simulink model "gm_UZ_EnDat"  (R2023b)
settings: Solver=FixedStepDiscrete  StartTime=0  StopTime=0.002  RelTol=1e-3
model workspace (MAT data in the model file):
  Select = 0
libraries: hdlsllib x314, hdlmdlgenlib x10, simulink x7, simulink_extras x3
(part 4 of 7)

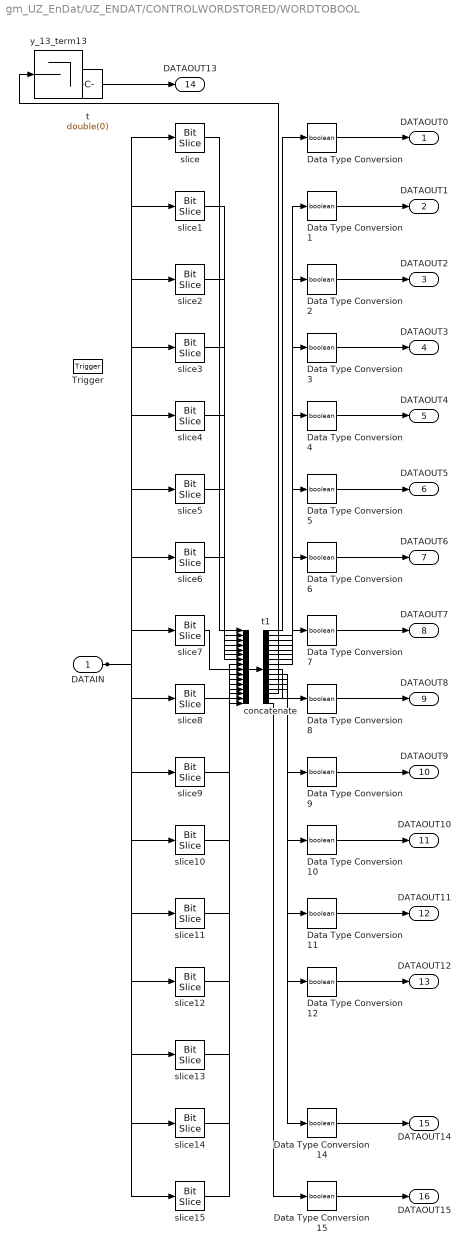
== system gm_UZ_EnDat/UZ_ENDAT/CONTROLWORDSTORED/WORDTOBOOL ==
  DATAIN : Inport  OutDataTypeStr=uint16  PortDimensions=1
  Trigger : TriggerPort  TriggerType=falling  VariantControl=(inherit)  OutputDataType=int8  InitialTriggerSignalState=positive  PortDimensions=1  OutDataTypeStr=boolean
  Data Type Conversion{,1..12,14..15} (15 alike) : DataTypeConversion  OutDataTypeStr=boolean  SaturateOnIntegerOverflow=off  RndMeth=Floor
  concatenate : Concatenate  NumInputs=16  Mode=Multidimensional array  ConcatenateDimension=2
  slice : hdlsllib/Logic and Bit Operations/Bit Slice  lidx=double(0)  ridx=double(0)
  slice1 : hdlsllib/Logic and Bit Operations/Bit Slice  lidx=double(1)  ridx=double(1)
  slice10 : hdlsllib/Logic and Bit Operations/Bit Slice  lidx=double(10)  ridx=double(10)
  slice11 : hdlsllib/Logic and Bit Operations/Bit Slice  lidx=double(11)  ridx=double(11)
  slice12 : hdlsllib/Logic and Bit Operations/Bit Slice  lidx=double(12)  ridx=double(12)
  slice13 : hdlsllib/Logic and Bit Operations/Bit Slice  lidx=double(13)  ridx=double(13)
  slice14 : hdlsllib/Logic and Bit Operations/Bit Slice  lidx=double(14)  ridx=double(14)
  slice15 : hdlsllib/Logic and Bit Operations/Bit Slice  lidx=double(15)  ridx=double(15)
  slice2 : hdlsllib/Logic and Bit Operations/Bit Slice  lidx=double(2)  ridx=double(2)
  slice3 : hdlsllib/Logic and Bit Operations/Bit Slice  lidx=double(3)  ridx=double(3)
  slice4 : hdlsllib/Logic and Bit Operations/Bit Slice  lidx=double(4)  ridx=double(4)
  slice5 : hdlsllib/Logic and Bit Operations/Bit Slice  lidx=double(5)  ridx=double(5)
  slice6 : hdlsllib/Logic and Bit Operations/Bit Slice  lidx=double(6)  ridx=double(6)
  slice7 : hdlsllib/Logic and Bit Operations/Bit Slice  lidx=double(7)  ridx=double(7)
  slice8 : hdlsllib/Logic and Bit Operations/Bit Slice  lidx=double(8)  ridx=double(8)
  slice9 : hdlsllib/Logic and Bit Operations/Bit Slice  lidx=double(9)  ridx=double(9)
  t : Constant  Value=double(0)  OutDataTypeStr=boolean  SampleTime=-1
  t1 : Demux  Outputs=16
  y_13_term13 : Terminator
  DATAOUT0 : Outport  InitialOutput=0
  DATAOUT1 : Outport  Port=2  InitialOutput=0
  DATAOUT2 : Outport  Port=3  InitialOutput=0
  DATAOUT3 : Outport  Port=4  InitialOutput=0
  DATAOUT4 : Outport  Port=5  InitialOutput=0
  DATAOUT5 : Outport  Port=6  InitialOutput=0
  DATAOUT6 : Outport  Port=7  InitialOutput=0
  DATAOUT7 : Outport  Port=8  InitialOutput=0
  DATAOUT8 : Outport  Port=9  InitialOutput=0
  DATAOUT9 : Outport  Port=10  InitialOutput=0
  DATAOUT10 : Outport  Port=11  InitialOutput=0
  DATAOUT11 : Outport  Port=12  InitialOutput=0
  DATAOUT12 : Outport  Port=13  InitialOutput=0
  DATAOUT13 : Outport  Port=14  InitialOutput=0
  DATAOUT14 : Outport  Port=15  InitialOutput=0
  DATAOUT15 : Outport  Port=16  InitialOutput=0
  wires:
  DATAIN/1 -> slice15/1, slice14/1, slice13/1, slice12/1, slice11/1, slice10/1, slice9/1, slice8/1, slice7/1, slice6/1, slice5/1, slice4/1, slice3/1, slice2/1, slice1/1, slice/1
  Data Type Conversion/1 -> DATAOUT0/1
  Data Type Conversion1/1 -> DATAOUT1/1
  Data Type Conversion10/1 -> DATAOUT10/1
  Data Type Conversion11/1 -> DATAOUT11/1
  Data Type Conversion12/1 -> DATAOUT12/1
  t/1 -> DATAOUT13/1
  Data Type Conversion14/1 -> DATAOUT14/1
  Data Type Conversion15/1 -> DATAOUT15/1
  Data Type Conversion2/1 -> DATAOUT2/1
  Data Type Conversion3/1 -> DATAOUT3/1
  Data Type Conversion4/1 -> DATAOUT4/1
  Data Type Conversion5/1 -> DATAOUT5/1
  Data Type Conversion6/1 -> DATAOUT6/1
  Data Type Conversion7/1 -> DATAOUT7/1
  Data Type Conversion8/1 -> DATAOUT8/1
  Data Type Conversion9/1 -> DATAOUT9/1
  concatenate/1 -> t1/1
  t1/1 -> Data Type Conversion/1
  t1/2 -> Data Type Conversion1/1
  t1/3 -> Data Type Conversion2/1
  t1/4 -> Data Type Conversion3/1
  t1/5 -> Data Type Conversion4/1
  t1/6 -> Data Type Conversion5/1
  t1/7 -> Data Type Conversion6/1
  t1/8 -> Data Type Conversion7/1
  t1/9 -> Data Type Conversion8/1
  t1/10 -> Data Type Conversion9/1
  t1/11 -> Data Type Conversion10/1
  t1/12 -> Data Type Conversion11/1
  t1/13 -> Data Type Conversion12/1
  t1/14 -> y_13_term13/1
  t1/15 -> Data Type Conversion14/1
  t1/16 -> Data Type Conversion15/1
  slice/1 -> concatenate/1
  slice1/1 -> concatenate/2
  slice2/1 -> concatenate/3
  slice3/1 -> concatenate/4
  slice4/1 -> concatenate/5
  slice5/1 -> concatenate/6
  slice6/1 -> concatenate/7
  slice7/1 -> concatenate/8
  slice8/1 -> concatenate/9
  slice9/1 -> concatenate/10
  slice10/1 -> concatenate/11
  slice11/1 -> concatenate/12
  slice12/1 -> concatenate/13
  slice13/1 -> concatenate/14
  slice14/1 -> concatenate/15
  slice15/1 -> concatenate/16

== system gm_UZ_EnDat/UZ_ENDAT/CRC_Check/DFF1 ==
  SET : Inport  OutDataTypeStr=boolean  PortDimensions=1  SampleTime=1e-08
  CLK : Inport  Port=2  OutDataTypeStr=boolean  PortDimensions=1  SampleTime=1e-08
  D : Inport  Port=3  OutDataTypeStr=boolean  PortDimensions=1  SampleTime=1e-08
  RST : Inport  Port=4  OutDataTypeStr=boolean  PortDimensions=1  SampleTime=1e-08
  JKFF : Subsystem
  NOT : Logic  Operator=NOT  Inputs=1  AllPortsSameDT=off  OutDataTypeStr=boolean  SampleTime=1e-08
  OQ : Outport  SampleTime=1e-08
  NOQ : Outport  Port=2  SampleTime=1e-08
  wires:
  SET/1 -> JKFF/1(SET)
  CLK/1 -> JKFF/2(CLK)
  D/1 -> NOT/1, JKFF/3(J)
  RST/1 -> JKFF/4(RST)
  JKFF/1(OQ) -> OQ/1
  JKFF/2(NOQ) -> NOQ/1
  NOT/1 -> JKFF/5(K)

== system gm_UZ_EnDat/UZ_ENDAT/CRC_Check/DFF2 ==
  SET : Inport  OutDataTypeStr=boolean  PortDimensions=1  SampleTime=1e-08
  CLK : Inport  Port=2  OutDataTypeStr=boolean  PortDimensions=1  SampleTime=1e-08
  D : Inport  Port=3  OutDataTypeStr=boolean  PortDimensions=1  SampleTime=1e-08
  RST : Inport  Port=4  OutDataTypeStr=boolean  PortDimensions=1  SampleTime=1e-08
  JKFF : Subsystem
  NOT : Logic  Operator=NOT  Inputs=1  AllPortsSameDT=off  OutDataTypeStr=boolean  SampleTime=1e-08
  OQ : Outport  SampleTime=1e-08
  NOQ : Outport  Port=2  SampleTime=1e-08
  wires:
  NOT/1 -> JKFF/5(K)
  JKFF/2(NOQ) -> NOQ/1
  JKFF/1(OQ) -> OQ/1
  RST/1 -> JKFF/4(RST)
  D/1 -> JKFF/3(J), NOT/1
  CLK/1 -> JKFF/2(CLK)
  SET/1 -> JKFF/1(SET)

== system gm_UZ_EnDat/UZ_ENDAT/CRC_Check/DFF3 ==
  SET : Inport  OutDataTypeStr=boolean  PortDimensions=1  SampleTime=1e-08
  CLK : Inport  Port=2  OutDataTypeStr=boolean  PortDimensions=1  SampleTime=1e-08
  D : Inport  Port=3  OutDataTypeStr=boolean  PortDimensions=1  SampleTime=1e-08
  RST : Inport  Port=4  OutDataTypeStr=boolean  PortDimensions=1  SampleTime=1e-08
  JKFF : Subsystem
  NOT : Logic  Operator=NOT  Inputs=1  AllPortsSameDT=off  OutDataTypeStr=boolean  SampleTime=1e-08
  OQ : Outport  SampleTime=1e-08
  NOQ : Outport  Port=2  SampleTime=1e-08
  wires:
  NOT/1 -> JKFF/5(K)
  JKFF/2(NOQ) -> NOQ/1
  JKFF/1(OQ) -> OQ/1
  RST/1 -> JKFF/4(RST)
  D/1 -> JKFF/3(J), NOT/1
  CLK/1 -> JKFF/2(CLK)
  SET/1 -> JKFF/1(SET)

== system gm_UZ_EnDat/UZ_ENDAT/CRC_Check/DFF4 ==
  SET : Inport  OutDataTypeStr=boolean  PortDimensions=1  SampleTime=1e-08
  CLK : Inport  Port=2  OutDataTypeStr=boolean  PortDimensions=1  SampleTime=1e-08
  D : Inport  Port=3  OutDataTypeStr=boolean  PortDimensions=1  SampleTime=1e-08
  RST : Inport  Port=4  OutDataTypeStr=boolean  PortDimensions=1  SampleTime=1e-08
  JKFF : Subsystem
  NOT : Logic  Operator=NOT  Inputs=1  AllPortsSameDT=off  OutDataTypeStr=boolean  SampleTime=1e-08
  OQ : Outport  SampleTime=1e-08
  NOQ : Outport  Port=2  SampleTime=1e-08
  wires:
  NOT/1 -> JKFF/5(K)
  JKFF/2(NOQ) -> NOQ/1
  JKFF/1(OQ) -> OQ/1
  RST/1 -> JKFF/4(RST)
  D/1 -> JKFF/3(J), NOT/1
  CLK/1 -> JKFF/2(CLK)
  SET/1 -> JKFF/1(SET)

== system gm_UZ_EnDat/UZ_ENDAT/CRC_Check/DFF5 ==
  SET : Inport  OutDataTypeStr=boolean  PortDimensions=1  SampleTime=1e-08
  CLK : Inport  Port=2  OutDataTypeStr=boolean  PortDimensions=1  SampleTime=1e-08
  D : Inport  Port=3  OutDataTypeStr=boolean  PortDimensions=1  SampleTime=1e-08
  RST : Inport  Port=4  OutDataTypeStr=boolean  PortDimensions=1  SampleTime=1e-08
  JKFF : Subsystem
  NOT : Logic  Operator=NOT  Inputs=1  AllPortsSameDT=off  OutDataTypeStr=boolean  SampleTime=1e-08
  OQ : Outport  SampleTime=1e-08
  NOQ : Outport  Port=2  SampleTime=1e-08
  wires:
  NOT/1 -> JKFF/5(K)
  JKFF/2(NOQ) -> NOQ/1
  JKFF/1(OQ) -> OQ/1
  RST/1 -> JKFF/4(RST)
  D/1 -> JKFF/3(J), NOT/1
  CLK/1 -> JKFF/2(CLK)
  SET/1 -> JKFF/1(SET)

== system gm_UZ_EnDat/UZ_ENDAT/INITIALOFF/CLKCNTER_FAST ==
  CLK : Inport  OutDataTypeStr=boolean  PortDimensions=1  SampleTime=1e-08
  Positional_Counter : Subsystem
  rd_0 : Delay  DelayLength=double(1)  InitialCondition=0  SampleTime=1e-08
  CNT : Outport  SampleTime=1e-08
  wires:
  Positional_Counter/1(divider) -> rd_0/1, CNT/1
  CLK/1 -> Positional_Counter/Trigger
  rd_0/1 -> Positional_Counter/1(valueout)

== system gm_UZ_EnDat/UZ_ENDAT/INITIALOFF/Subsystem6 ==
  FACTOR : Inport  OutMin=0  OutMax=60000  OutDataTypeStr=uint16  PortDimensions=1  SampleTime=1e-08
  Add1 : Sum  Inputs=+-  OutDataTypeStr=uint16  AccumDataTypeStr=fixdt(1, 17, 0)  RndMeth=Simplest  SaturateOnIntegerOverflow=on  SampleTime=1e-08
  Add2 : Sum  OutDataTypeStr=uint16  AccumDataTypeStr=fixdt(1, 33, 0)  RndMeth=Simplest  SaturateOnIntegerOverflow=on  SampleTime=1e-08
  Add3 : Sum  Inputs=+-  OutDataTypeStr=uint16  AccumDataTypeStr=fixdt(1, 17, 0)  RndMeth=Simplest  SaturateOnIntegerOverflow=on  SampleTime=1e-08
  Compare To Constant : Subsystem  mask(Compare To Constant){relop=<, const=double(100), OutDataTypeStr=boolean, ZeroCross=on}
      mask prompts: relop "Simulink:masks:Operator_MP"; const "Simulink:masks:ConstantValue_MP"; OutDataTypeStr "Simulink:masks:OutputDataType_MP"; ZeroCross "Simulink:masks:EnableZerocrossingDetection_MP"
      mask help: Simulink:masks:CompareToConstant_MD
      mask TypeOptions relop: == | ~= | < | <= | >= | >
      mask TypeOptions OutDataTypeStr: Simulink:masks:uint8 | Simulink:masks:boolean
      mask Callback ZeroCross: sl('zeroCrossEnable', gcbh);
      mask Display: disp(str)
  Constant : Constant  Value=20  OutDataTypeStr=int16  SampleTime=1e-08
  Constant1 : Constant  Value=-20  OutDataTypeStr=int16  SampleTime=1e-08
  Constant2 : Constant  Value=100  OutDataTypeStr=uint16  SampleTime=1e-08
  Constant3 : Constant  Value=2000  OutDataTypeStr=uint16  SampleTime=1e-08
  HwModeRegister : Delay  DelayLength=double(1)  InitialCondition=0  SampleTime=1e-08
  HwModeRegister1 : Delay  DelayLength=double(1)  InitialCondition=0  SampleTime=1e-08
  PipelineRegister : Delay  DelayLength=double(1)  InitialCondition=0  SampleTime=1e-08
  Product : Product  Inputs=**  OutDataTypeStr=int32  SampleTime=1e-08
  Switch : Switch  Criteria=u2 > Threshold  Threshold=double(0)  OutDataTypeStr=uint16  SampleTime=1e-08  SaturateOnIntegerOverflow=off  InputSameDT=off
  Switch1 : Switch  Criteria=u2 > Threshold  Threshold=double(0)  OutDataTypeStr=int16  SampleTime=1e-08  SaturateOnIntegerOverflow=off  InputSameDT=off
  out : Outport  SampleTime=1e-08
  wires:
  FACTOR/1 -> Add3/1, Add1/2, Compare To Constant/1(u)
  Add1/1 -> Switch/1
  Add2/1 -> out/1
  Add3/1 -> Switch/3
  Compare To Constant/1(y) -> Switch1/2, Switch/2
  Constant/1 -> Switch1/3
  Constant1/1 -> Switch1/1
  Constant2/1 -> Add3/2, Add1/1
  Constant3/1 -> Add2/1
  PipelineRegister/1 -> Add2/2
  Switch/1 -> HwModeRegister/1
  Switch1/1 -> HwModeRegister1/1
  Product/1 -> PipelineRegister/1
  HwModeRegister/1 -> Product/1
  HwModeRegister1/1 -> Product/2

== system gm_UZ_EnDat/UZ_ENDAT/ManualSerialize/Compare To Constant ==
  u : Inport  OutDataTypeStr=uint8  SampleTime=1e-08
  Compare : RelationalOperator  Operator===  OutDataTypeStr=boolean
  Constant : Constant  DisableCoverage=on  Value=const  OutDataTypeStr=Inherit: Inherit via back propagation  SampleTime=-1
  y : Outport  SampleTime=1e-08
  wires:
  u/1 -> Compare/1
  Compare/1 -> y/1
  Constant/1 -> Compare/2

== system gm_UZ_EnDat/UZ_ENDAT/ManualSerialize/Detect Increase1 ==
  note: U(k)
  note: Edge
  U : Inport  OutDataTypeStr=boolean  SampleTime=1e-08
  FixPt Relational Operator : RelationalOperator  Operator=>  OutDataTypeStr=boolean  SampleTime=1e-08  InputSameDT=off
  rd_0 : Delay  DelayLength=double(1)  InitialCondition=0  SampleTime=1e-08
  t : hdlmdlgenlib/Buffer
  Y : Outport  SampleTime=1e-08
  wires:
  U/1 -> t/1, FixPt Relational Operator/1
  t/1 -> rd_0/1
  FixPt Relational Operator/1 -> Y/1
  rd_0/1 -> FixPt Relational Operator/2

== system gm_UZ_EnDat/UZ_ENDAT/ManualSerialize/FF1 ==
  SET : Inport  OutDataTypeStr=boolean  PortDimensions=1  SampleTime=1e-08
  RST : Inport  Port=2  OutDataTypeStr=boolean  PortDimensions=1  SampleTime=1e-08
  S-R Flip-Flop : simulink_extras/Flip Flops/S-R Flip-Flop  initial_condition=0
  OQ : Outport  SampleTime=1e-08
  NOQ : Outport  Port=2  SampleTime=1e-08
  wires:
  SET/1 -> S-R Flip-Flop/1
  RST/1 -> S-R Flip-Flop/2
  S-R Flip-Flop/1 -> OQ/1
  S-R Flip-Flop/2 -> NOQ/1

== system gm_UZ_EnDat/UZ_ENDAT/ManualSerialize/SetZero64modified ==
  valin : Inport  OutDataTypeStr=fixdt(0, 64, 0)  PortDimensions=1
  setzero : Inport  Port=2  OutDataTypeStr=boolean  PortDimensions=1
  Trigger : TriggerPort  TriggerType=either  VariantControl=(inherit)  PortDimensions=1  OutDataTypeStr=boolean
  Constant2 : Constant  Value="fi(0,0,64,0,\"hex\",\"0000000000000000\")"  OutDataTypeStr=fixdt(0, 64, 0)  SampleTime=-1
  Index Vector1 : MultiPortSwitch  DataPortOrder=Zero-based contiguous  Inputs=2  DiagnosticForDefault=None  zeroidx=on  OutDataTypeStr=fixdt(0, 64, 0)  SaturateOnIntegerOverflow=off  InputSameDT=off
  valueout : Outport  InitialOutput=0  VectorParamsAs1DForOutWhenUnconnected=off
  wires:
  valin/1 -> Index Vector1/2
  setzero/1 -> Index Vector1/1
  Constant2/1 -> Index Vector1/3
  Index Vector1/1 -> valueout/1

== system gm_UZ_EnDat/UZ_ENDAT/ManualSerialize/Storage1 ==
  Data : Inport  OutDataTypeStr=fixdt(0, 64, 0)  PortDimensions=1  SampleTime=1e-08
  Write : Inport  Port=2  OutDataTypeStr=boolean  PortDimensions=1  SampleTime=1e-08
  Compare To Zero : Subsystem  mask(Compare To Zero){relop=>, OutDataTypeStr=boolean, ZeroCross=on}
      mask prompts: relop "Simulink:masks:Operator_MP"; OutDataTypeStr "Simulink:masks:OutputDataType_MP"; ZeroCross "Simulink:masks:EnableZerocrossingDetection_MP"
      mask help: Simulink:masks:CompareToZero_MD
      mask TypeOptions relop: == | ~= | < | <= | >= | >
      mask TypeOptions OutDataTypeStr: Simulink:masks:uint8 | Simulink:masks:boolean
      mask Callback ZeroCross: sl('zeroCrossEnable', gcbh);
      mask Display: disp([relop,' 0'])
  Logical Operator1 : Logic  AllPortsSameDT=off  OutDataTypeStr=boolean  SampleTime=1e-08
  out : Outport  SampleTime=1e-08
  wrok : Outport  Port=2  OutDataTypeStr=boolean  SampleTime=1e-08
  wires:
  Data/1 -> out/1, Compare To Zero/1(u)
  Write/1 -> Logical Operator1/1
  Compare To Zero/1(y) -> Logical Operator1/2
  Logical Operator1/1 -> wrok/1

== system gm_UZ_EnDat/UZ_ENDAT/ManualSerialize/Subsystem ==
  countclk : Inport  OutDataTypeStr=boolean  PortDimensions=1  SampleTime=1e-08
  reset : Inport  Port=2  OutDataTypeStr=boolean  PortDimensions=1  SampleTime=1e-08
  Detect Increase : Subsystem  mask(Detect Increase){vinit=double(0), InputProcessing=Elements as channels (sample based), OutDataTypeStr=boolean}
      mask prompts: vinit "Simulink:masks:InitialCondition_MP"; InputProcessing "Simulink:masks:InputProcessing_MP"; OutDataTypeStr "Simulink:masks:OutputDataType_MP"
      mask help: Simulink:masks:DetectIncrease_MD
      mask TypeOptions InputProcessing: Simulink:masks:ColumnsAsChannelsFrameBased | Simulink:masks:ElementsAsChannelsSampleBased
      mask TypeOptions OutDataTypeStr: Simulink:masks:uint8 | Simulink:masks:boolean
      mask Display: fprintf('U > U/z')
  HDL Counter_enbsw : Switch  Criteria=u2 ~= 0  Threshold=double(0)  OutDataTypeStr=uint8  SampleTime=1e-08  SaturateOnIntegerOverflow=off  InputSameDT=off
  adder : Sum  OutDataTypeStr=uint8  AccumDataTypeStr=uint8  SampleTime=1e-08
  compare : simulink/Logic and Bit Operations/Compare To Constant  relop===  const="fi(0,0,8,0,\"hex\",\"33\")"  OutDataTypeStr=boolean
  const : Constant  Value=0  VectorParams1D=off  OutDataTypeStr=uint8  SampleTime=1e-08
  countFrom : Constant  Value=0  VectorParams1D=off  OutDataTypeStr=uint8  SampleTime=1e-08
  rd_0 : Delay  DelayLength=double(1)  InitialCondition=0  SampleTime=1e-08
  rd_1 : Delay  DelayLength=double(2)  InitialCondition=0  SampleTime=1e-08
  rd_2 : Delay  DelayLength=double(1)  InitialCondition=0  SampleTime=1e-08
  stateControl : Constant  OutDataTypeStr=boolean  SampleTime=1e-08
  step_value : Constant  VectorParams1D=off  OutDataTypeStr=uint8  SampleTime=1e-08
  switch : Switch  Criteria=u2 ~= 0  Threshold=double(0)  OutDataTypeStr=uint8  SampleTime=1e-08  SaturateOnIntegerOverflow=off  InputSameDT=off
  switchEnable : MultiPortSwitch  DataPortOrder=Zero-based contiguous  Inputs=2  DiagnosticForDefault=None  zeroidx=on  OutDataTypeStr=uint8  SampleTime=1e-08  SaturateOnIntegerOverflow=off  InputSameDT=off
  switchReset : Switch  Criteria=u2 ~= 0  Threshold=double(0)  OutDataTypeStr=uint8  SampleTime=1e-08  SaturateOnIntegerOverflow=off  InputSameDT=off
  valin1 : Outport  SampleTime=1e-08  InitialOutput=0
  wires:
  countclk/1 -> Detect Increase/1(U)
  reset/1 -> rd_0/1
  stateControl/1 -> rd_1/1
  step_value/1 -> adder/2
  countFrom/1 -> switch/1
  Detect Increase/1(Y) -> switchEnable/1
  const/1 -> switchReset/1
  adder/1 -> switch/3
  compare/1 -> switch/2
  switch/1 -> switchEnable/3
  switchEnable/1 -> switchReset/3
  switchReset/1 -> HDL Counter_enbsw/1
  rd_0/1 -> switchReset/2
  rd_1/1 -> HDL Counter_enbsw/2
  HDL Counter_enbsw/1 -> rd_2/1
  rd_2/1 -> HDL Counter_enbsw/3, adder/1, compare/1, switchEnable/2, valin1/1

== system gm_UZ_EnDat/UZ_ENDAT/ManualSerialize/Triggered Subsystem ==
  DATA : Inport  OutDataTypeStr=boolean  PortDimensions=1
  valueout : Inport  Port=2  OutDataTypeStr=fixdt(0, 64, 0)  PortDimensions=1
  Trigger : TriggerPort  VariantControl=(inherit)  PortDimensions=1  OutDataTypeStr=boolean
  Bit Clear : simulink/Logic and Bit Operations/Bit Clear  iBit=double(50)
  Bit Set : simulink/Logic and Bit Operations/Bit Set  iBit=double(50)
  Bit Shift : hdlsllib/Logic and Bit Operations/Bit Shift  mode=Shift Right Logical  N=double(1)
  Switch : Switch  Criteria=u2 ~= 0  Threshold=double(0)  OutDataTypeStr=fixdt(0, 64, 0)  SaturateOnIntegerOverflow=off  InputSameDT=off
  valin : Outport  InitialOutput=0
  wires:
  DATA/1 -> Switch/2
  valueout/1 -> Bit Set/1, Bit Clear/1
  Bit Clear/1 -> Switch/3
  Bit Set/1 -> Switch/1
  Bit Shift/1 -> valin/1
  Switch/1 -> Bit Shift/1

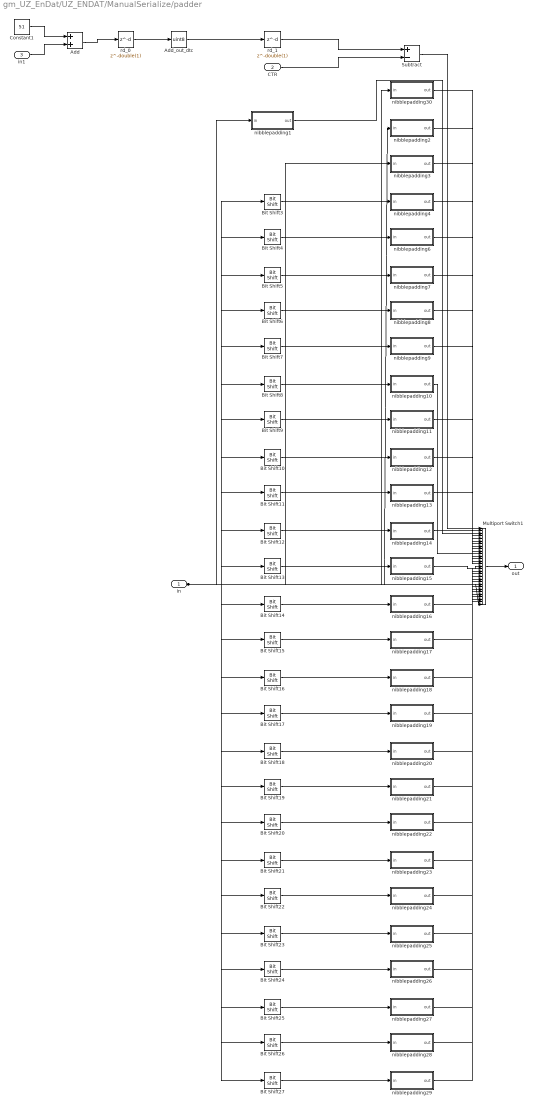
== system gm_UZ_EnDat/UZ_ENDAT/ManualSerialize/padder ==
  in : Inport  OutDataTypeStr=fixdt(0, 64, 0)  PortDimensions=1  SampleTime=1e-08
  CTR : Inport  Port=2  OutDataTypeStr=uint8  PortDimensions=1  SampleTime=1e-08
  in1 : Inport  Port=3  OutDataTypeStr=int8  PortDimensions=1  SampleTime=1e-08
  Add : Sum  OutDataTypeStr=fixdt(1, 10, 0)  AccumDataTypeStr=fixdt(1, 10, 0)  SampleTime=1e-08
  Add_out_dtc : DataTypeConversion  OutDataTypeStr=uint8  RndMeth=Simplest  SampleTime=1e-08  SaturateOnIntegerOverflow=off
  Bit Shift10 : hdlsllib/Logic and Bit Operations/Bit Shift  mode=Shift Right Logical  N=double(8)
  Bit Shift11 : hdlsllib/Logic and Bit Operations/Bit Shift  mode=Shift Right Logical  N=double(9)
  Bit Shift12 : hdlsllib/Logic and Bit Operations/Bit Shift  mode=Shift Right Logical  N=double(10)
  Bit Shift13 : hdlsllib/Logic and Bit Operations/Bit Shift  mode=Shift Right Logical  N=double(11)
  Bit Shift14 : hdlsllib/Logic and Bit Operations/Bit Shift  mode=Shift Right Logical  N=double(12)
  Bit Shift15 : hdlsllib/Logic and Bit Operations/Bit Shift  mode=Shift Right Logical  N=double(13)
  Bit Shift16 : hdlsllib/Logic and Bit Operations/Bit Shift  mode=Shift Right Logical  N=double(14)
  Bit Shift17 : hdlsllib/Logic and Bit Operations/Bit Shift  mode=Shift Right Logical  N=double(15)
  Bit Shift18 : hdlsllib/Logic and Bit Operations/Bit Shift  mode=Shift Right Logical  N=double(16)
  Bit Shift19 : hdlsllib/Logic and Bit Operations/Bit Shift  mode=Shift Right Logical  N=double(17)
  Bit Shift20 : hdlsllib/Logic and Bit Operations/Bit Shift  mode=Shift Right Logical  N=double(18)
  Bit Shift21 : hdlsllib/Logic and Bit Operations/Bit Shift  mode=Shift Right Logical  N=double(19)
  Bit Shift22 : hdlsllib/Logic and Bit Operations/Bit Shift  mode=Shift Right Logical  N=double(20)
  Bit Shift23 : hdlsllib/Logic and Bit Operations/Bit Shift  mode=Shift Right Logical  N=double(21)
  Bit Shift24 : hdlsllib/Logic and Bit Operations/Bit Shift  mode=Shift Right Logical  N=double(22)
  Bit Shift25 : hdlsllib/Logic and Bit Operations/Bit Shift  mode=Shift Right Logical  N=double(23)
  Bit Shift26 : hdlsllib/Logic and Bit Operations/Bit Shift  mode=Shift Right Logical  N=double(24)
  Bit Shift27 : hdlsllib/Logic and Bit Operations/Bit Shift  mode=Shift Right Logical  N=double(25)
  Bit Shift3 : hdlsllib/Logic and Bit Operations/Bit Shift  mode=Shift Right Logical  N=double(1)
  Bit Shift4 : hdlsllib/Logic and Bit Operations/Bit Shift  mode=Shift Right Logical  N=double(2)
  Bit Shift5 : hdlsllib/Logic and Bit Operations/Bit Shift  mode=Shift Right Logical  N=double(3)
  Bit Shift6 : hdlsllib/Logic and Bit Operations/Bit Shift  mode=Shift Right Logical  N=double(4)
  Bit Shift7 : hdlsllib/Logic and Bit Operations/Bit Shift  mode=Shift Right Logical  N=double(5)
  Bit Shift8 : hdlsllib/Logic and Bit Operations/Bit Shift  mode=Shift Right Logical  N=double(6)
  Bit Shift9 : hdlsllib/Logic and Bit Operations/Bit Shift  mode=Shift Right Logical  N=double(7)
  Constant1 : Constant  Value=51  OutDataTypeStr=uint8  SampleTime=1e-08
  Multiport Switch1 : MultiPortSwitch  DataPortOrder=Zero-based contiguous  Inputs=29  DataPortForDefault=Additional data port  DiagnosticForDefault=None  zeroidx=on  OutDataTypeStr=fixdt(0, 64, 0)  RndMeth=Simplest  SampleTime=1e-08  SaturateOnIntegerOverflow=off  InputSameDT=off
  Subtract : Sum  Inputs=+-  OutDataTypeStr=uint8  AccumDataTypeStr=fixdt(1, 9, 0)  RndMeth=Simplest  SaturateOnIntegerOverflow=on  SampleTime=1e-08
  nibblepadding1 : Subsystem
  nibblepadding10 : Subsystem
  nibblepadding11 : Subsystem
  nibblepadding12 : Subsystem
  nibblepadding13 : Subsystem
  nibblepadding14 : Subsystem
  nibblepadding15 : Subsystem
  nibblepadding16 : Subsystem
  nibblepadding17 : Subsystem
  nibblepadding18 : Subsystem
  nibblepadding19 : Subsystem
  nibblepadding2 : Subsystem
  nibblepadding20 : Subsystem
  nibblepadding21 : Subsystem
  nibblepadding22 : Subsystem
  nibblepadding23 : Subsystem
  nibblepadding24 : Subsystem
  nibblepadding25 : Subsystem
  nibblepadding26 : Subsystem
  nibblepadding27 : Subsystem
  nibblepadding28 : Subsystem
  nibblepadding29 : Subsystem
  nibblepadding3 : Subsystem
  nibblepadding30 : Subsystem
  nibblepadding4 : Subsystem
  nibblepadding6 : Subsystem
  nibblepadding7 : Subsystem
  nibblepadding8 : Subsystem
  nibblepadding9 : Subsystem
  rd_0 : Delay  DelayLength=double(1)  InitialCondition=0  SampleTime=1e-08
  rd_1 : Delay  DelayLength=double(1)  InitialCondition=0  SampleTime=1e-08
  out : Outport  SampleTime=1e-08
  wires:
  in/1 -> Multiport Switch1/31, Bit Shift9/1, Bit Shift8/1, Bit Shift7/1, Bit Shift6/1, Bit Shift5/1, Bit Shift4/1, Bit Shift3/1, Bit Shift27/1, Bit Shift26/1, Bit Shift25/1, Bit Shift24/1, Bit Shift23/1, Bit Shift22/1, Bit Shift21/1, Bit Shift20/1, Bit Shift19/1, Bit Shift18/1, Bit Shift17/1, Bit Shift16/1, Bit Shift15/1, Bit Shift14/1, Bit Shift13/1, Bit Shift12/1, Bit Shift11/1, Bit Shift10/1, nibblepadding1/1(in), nibblepadding2/1(in), nibblepadding3/1(in), nibblepadding30/1(in)
  CTR/1 -> Subtract/2
  in1/1 -> Add/2
  Bit Shift10/1 -> nibblepadding12/1(in)
  Bit Shift11/1 -> nibblepadding13/1(in)
  Bit Shift12/1 -> nibblepadding14/1(in)
  Bit Shift13/1 -> nibblepadding15/1(in)
  Bit Shift14/1 -> nibblepadding16/1(in)
  Bit Shift15/1 -> nibblepadding17/1(in)
  Bit Shift16/1 -> nibblepadding18/1(in)
  Bit Shift17/1 -> nibblepadding19/1(in)
  Bit Shift18/1 -> nibblepadding20/1(in)
  Bit Shift19/1 -> nibblepadding21/1(in)
  Bit Shift20/1 -> nibblepadding22/1(in)
  Bit Shift21/1 -> nibblepadding23/1(in)
  Bit Shift22/1 -> nibblepadding24/1(in)
  Bit Shift23/1 -> nibblepadding25/1(in)
  Bit Shift24/1 -> nibblepadding26/1(in)
  Bit Shift25/1 -> nibblepadding27/1(in)
  Bit Shift26/1 -> nibblepadding28/1(in)
  Bit Shift27/1 -> nibblepadding29/1(in)
  Bit Shift3/1 -> nibblepadding4/1(in)
  Bit Shift4/1 -> nibblepadding6/1(in)
  Bit Shift5/1 -> nibblepadding7/1(in)
  Bit Shift6/1 -> nibblepadding8/1(in)
  Bit Shift7/1 -> nibblepadding9/1(in)
  Bit Shift8/1 -> nibblepadding10/1(in)
  Bit Shift9/1 -> nibblepadding11/1(in)
  Constant1/1 -> Add/1
  Multiport Switch1/1 -> out/1
  Subtract/1 -> Multiport Switch1/1
  nibblepadding1/1(out) -> Multiport Switch1/3
  nibblepadding10/1(out) -> Multiport Switch1/11
  nibblepadding11/1(out) -> Multiport Switch1/12
  nibblepadding12/1(out) -> Multiport Switch1/13
  nibblepadding13/1(out) -> Multiport Switch1/14
  nibblepadding14/1(out) -> Multiport Switch1/15
  nibblepadding15/1(out) -> Multiport Switch1/16
  nibblepadding16/1(out) -> Multiport Switch1/17
  nibblepadding17/1(out) -> Multiport Switch1/18
  nibblepadding18/1(out) -> Multiport Switch1/19
  nibblepadding19/1(out) -> Multiport Switch1/20
  nibblepadding2/1(out) -> Multiport Switch1/4
  nibblepadding20/1(out) -> Multiport Switch1/21
  nibblepadding21/1(out) -> Multiport Switch1/22
  nibblepadding22/1(out) -> Multiport Switch1/23
  nibblepadding23/1(out) -> Multiport Switch1/24
  nibblepadding24/1(out) -> Multiport Switch1/25
  nibblepadding25/1(out) -> Multiport Switch1/26
  nibblepadding26/1(out) -> Multiport Switch1/27
  nibblepadding27/1(out) -> Multiport Switch1/28
  nibblepadding28/1(out) -> Multiport Switch1/29
  nibblepadding29/1(out) -> Multiport Switch1/30
  nibblepadding3/1(out) -> Multiport Switch1/5
  nibblepadding30/1(out) -> Multiport Switch1/2
  nibblepadding4/1(out) -> Multiport Switch1/6
  nibblepadding6/1(out) -> Multiport Switch1/7
  nibblepadding7/1(out) -> Multiport Switch1/8
  nibblepadding8/1(out) -> Multiport Switch1/9
  nibblepadding9/1(out) -> Multiport Switch1/10
  Add/1 -> rd_0/1
  Add_out_dtc/1 -> rd_1/1
  rd_1/1 -> Subtract/1
  rd_0/1 -> Add_out_dtc/1

== system gm_UZ_EnDat/UZ_ENDAT/RESPONSESLICER3X/19BITSLICER ==
  DATA : Inport  OutDataTypeStr=fixdt(0, 64, 0)  PortDimensions=1  SampleTime=1e-08
  DATA1 : Inport  Port=2  OutDataTypeStr=fixdt(0, 64, 0)  PortDimensions=1  SampleTime=1e-08
  DATA2 : Inport  Port=3  OutDataTypeStr=fixdt(0, 64, 0)  PortDimensions=1  SampleTime=1e-08
  Enable : EnablePort  OutDataTypeStr=boolean
  responseslicer : Subsystem
  responseslicer1 : Subsystem
  responseslicer1_term2 : Terminator
  responseslicer2 : Subsystem
  responseslicer2_term2 : Terminator
  CRC : Outport  SampleTime=1e-08  InitialOutput=0
  payload : Outport  Port=2  SampleTime=1e-08  InitialOutput=0
  CRC1 : Outport  Port=3  SampleTime=1e-08  InitialOutput=0
  payload1 : Outport  Port=4  SampleTime=1e-08  InitialOutput=0
  CRC2 : Outport  Port=5  SampleTime=1e-08  InitialOutput=0
  payload2 : Outport  Port=6  SampleTime=1e-08  InitialOutput=0
  sensorerror : Outport  Port=7  SampleTime=1e-08  InitialOutput=0
  wires:
  DATA/1 -> responseslicer/1(DATA)
  DATA1/1 -> responseslicer1/1(DATA)
  DATA2/1 -> responseslicer2/1(DATA)
  responseslicer/1(CRC) -> CRC/1
  responseslicer/2(payload) -> payload/1
  responseslicer/3(error) -> sensorerror/1
  responseslicer1/1(CRC) -> CRC1/1
  responseslicer1/2(payload) -> payload1/1
  responseslicer1/3(error) -> responseslicer1_term2/1
  responseslicer2/1(CRC) -> CRC2/1
  responseslicer2/2(payload) -> payload2/1
  responseslicer2/3(error) -> responseslicer2_term2/1

== system gm_UZ_EnDat/UZ_ENDAT/RESPONSESLICER3X/21BITSLICER ==
  DATA : Inport  OutDataTypeStr=fixdt(0, 64, 0)  PortDimensions=1  SampleTime=1e-08
  DATA1 : Inport  Port=2  OutDataTypeStr=fixdt(0, 64, 0)  PortDimensions=1  SampleTime=1e-08
  DATA2 : Inport  Port=3  OutDataTypeStr=fixdt(0, 64, 0)  PortDimensions=1  SampleTime=1e-08
  Enable : EnablePort  OutDataTypeStr=boolean
  responseslicer : Subsystem
  responseslicer3 : Subsystem
  responseslicer3_term2 : Terminator
  responseslicer4 : Subsystem
  responseslicer4_term2 : Terminator
  CRC : Outport  SampleTime=1e-08  InitialOutput=0
  payload : Outport  Port=2  SampleTime=1e-08  InitialOutput=0
  CRC1 : Outport  Port=3  SampleTime=1e-08  InitialOutput=0
  payload1 : Outport  Port=4  SampleTime=1e-08  InitialOutput=0
  CRC2 : Outport  Port=5  SampleTime=1e-08  InitialOutput=0
  payload2 : Outport  Port=6  SampleTime=1e-08  InitialOutput=0
  sensorerror : Outport  Port=7  SampleTime=1e-08  InitialOutput=0
  wires:
  DATA/1 -> responseslicer/1(DATA)
  DATA1/1 -> responseslicer4/1(DATA)
  DATA2/1 -> responseslicer3/1(DATA)
  responseslicer/1(CRC) -> CRC/1
  responseslicer/2(payload) -> payload/1
  responseslicer/3(error) -> sensorerror/1
  responseslicer3/1(CRC) -> CRC2/1
  responseslicer3/2(payload) -> payload2/1
  responseslicer3/3(error) -> responseslicer3_term2/1
  responseslicer4/1(CRC) -> CRC1/1
  responseslicer4/2(payload) -> payload1/1
  responseslicer4/3(error) -> responseslicer4_term2/1

== system gm_UZ_EnDat/UZ_ENDAT/RESPONSESLICER3X/23BITSLICER ==
  DATA : Inport  OutDataTypeStr=fixdt(0, 64, 0)  PortDimensions=1  SampleTime=1e-08
  DATA1 : Inport  Port=2  OutDataTypeStr=fixdt(0, 64, 0)  PortDimensions=1  SampleTime=1e-08
  DATA2 : Inport  Port=3  OutDataTypeStr=fixdt(0, 64, 0)  PortDimensions=1  SampleTime=1e-08
  Enable : EnablePort  OutDataTypeStr=boolean
  responseslicer : Subsystem
  responseslicer1 : Subsystem
  responseslicer1_term2 : Terminator
  responseslicer2 : Subsystem
  responseslicer2_term2 : Terminator
  CRC : Outport  SampleTime=1e-08  InitialOutput=0
  payload : Outport  Port=2  SampleTime=1e-08  InitialOutput=0
  CRC1 : Outport  Port=3  SampleTime=1e-08  InitialOutput=0
  payload1 : Outport  Port=4  SampleTime=1e-08  InitialOutput=0
  CRC2 : Outport  Port=5  SampleTime=1e-08  InitialOutput=0
  payload2 : Outport  Port=6  SampleTime=1e-08  InitialOutput=0
  sensorerror : Outport  Port=7  SampleTime=1e-08  InitialOutput=0
  wires:
  DATA/1 -> responseslicer/1(DATA)
  DATA1/1 -> responseslicer1/1(DATA)
  DATA2/1 -> responseslicer2/1(DATA)
  responseslicer/1(CRC) -> CRC/1
  responseslicer/2(payload) -> payload/1
  responseslicer/3(error) -> sensorerror/1
  responseslicer1/1(CRC) -> CRC1/1
  responseslicer1/2(payload) -> payload1/1
  responseslicer1/3(error) -> responseslicer1_term2/1
  responseslicer2/1(CRC) -> CRC2/1
  responseslicer2/2(payload) -> payload2/1
  responseslicer2/3(error) -> responseslicer2_term2/1

== system gm_UZ_EnDat/UZ_ENDAT/RESPONSESLICER3X/25BITSLICER ==
  DATA : Inport  OutDataTypeStr=fixdt(0, 64, 0)  PortDimensions=1  SampleTime=1e-08
  DATA1 : Inport  Port=2  OutDataTypeStr=fixdt(0, 64, 0)  PortDimensions=1  SampleTime=1e-08
  DATA2 : Inport  Port=3  OutDataTypeStr=fixdt(0, 64, 0)  PortDimensions=1  SampleTime=1e-08
  Enable : EnablePort  OutDataTypeStr=boolean
  responseslicer : Subsystem
  responseslicer1 : Subsystem
  responseslicer1_term2 : Terminator
  responseslicer2 : Subsystem
  responseslicer2_term2 : Terminator
  CRC : Outport  SampleTime=1e-08  InitialOutput=0
  payload : Outport  Port=2  SampleTime=1e-08  InitialOutput=0
  CRC1 : Outport  Port=3  SampleTime=1e-08  InitialOutput=0
  payload1 : Outport  Port=4  SampleTime=1e-08  InitialOutput=0
  CRC2 : Outport  Port=5  SampleTime=1e-08  InitialOutput=0
  payload2 : Outport  Port=6  SampleTime=1e-08  InitialOutput=0
  sensorerror : Outport  Port=7  SampleTime=1e-08  InitialOutput=0
  wires:
  DATA/1 -> responseslicer/1(DATA)
  DATA1/1 -> responseslicer1/1(DATA)
  DATA2/1 -> responseslicer2/1(DATA)
  responseslicer/1(CRC) -> CRC/1
  responseslicer/2(payload) -> payload/1
  responseslicer/3(error) -> sensorerror/1
  responseslicer1/1(CRC) -> CRC1/1
  responseslicer1/2(payload) -> payload1/1
  responseslicer1/3(error) -> responseslicer1_term2/1
  responseslicer2/1(CRC) -> CRC2/1
  responseslicer2/2(payload) -> payload2/1
  responseslicer2/3(error) -> responseslicer2_term2/1

== system gm_UZ_EnDat/UZ_ENDAT/RESPONSESLICER3X/27BITSLICER ==
  DATA : Inport  OutDataTypeStr=fixdt(0, 64, 0)  PortDimensions=1  SampleTime=1e-08
  DATA1 : Inport  Port=2  OutDataTypeStr=fixdt(0, 64, 0)  PortDimensions=1  SampleTime=1e-08
  DATA2 : Inport  Port=3  OutDataTypeStr=fixdt(0, 64, 0)  PortDimensions=1  SampleTime=1e-08
  Enable : EnablePort  OutDataTypeStr=boolean
  responseslicer : Subsystem
  responseslicer1 : Subsystem
  responseslicer1_term2 : Terminator
  responseslicer2 : Subsystem
  responseslicer2_term2 : Terminator
  CRC : Outport  SampleTime=1e-08  InitialOutput=0
  payload : Outport  Port=2  SampleTime=1e-08  InitialOutput=0
  CRC1 : Outport  Port=3  SampleTime=1e-08  InitialOutput=0
  payload1 : Outport  Port=4  SampleTime=1e-08  InitialOutput=0
  CRC2 : Outport  Port=5  SampleTime=1e-08  InitialOutput=0
  payload2 : Outport  Port=6  SampleTime=1e-08  InitialOutput=0
  sensorerror : Outport  Port=7  SampleTime=1e-08  InitialOutput=0
  wires:
  DATA/1 -> responseslicer/1(DATA)
  DATA1/1 -> responseslicer1/1(DATA)
  DATA2/1 -> responseslicer2/1(DATA)
  responseslicer/1(CRC) -> CRC/1
  responseslicer/2(payload) -> payload/1
  responseslicer/3(error) -> sensorerror/1
  responseslicer1/1(CRC) -> CRC1/1
  responseslicer1/2(payload) -> payload1/1
  responseslicer1/3(error) -> responseslicer1_term2/1
  responseslicer2/1(CRC) -> CRC2/1
  responseslicer2/2(payload) -> payload2/1
  responseslicer2/3(error) -> responseslicer2_term2/1

== system gm_UZ_EnDat/UZ_ENDAT/Storage16/Compare To Zero ==
  u : Inport  OutDataTypeStr=uint16  SampleTime=1e-08
  Compare : RelationalOperator  Operator===  OutDataTypeStr=boolean  SampleTime=1e-08
  Constant : Constant  Value=0  OutDataTypeStr=uint16  SampleTime=1e-08
  y : Outport  SampleTime=1e-08
  wires:
  u/1 -> Compare/1
  Compare/1 -> y/1
  Constant/1 -> Compare/2

== system gm_UZ_EnDat/UZ_ENDAT/Subsystem2/ManualDeserializere ==
  CLK : Inport  OutDataTypeStr=boolean  PortDimensions=1  SampleTime=1e-08
  SLOWCLCK : Inport  Port=2  OutDataTypeStr=boolean  PortDimensions=1  SampleTime=1e-08
  DATA : Inport  Port=3  OutDataTypeStr=uint16  PortDimensions=1  SampleTime=1e-08
  reset : Inport  Port=4  OutDataTypeStr=boolean  PortDimensions=1  SampleTime=1e-08
  Constant3 : Constant  Value=0  OutDataTypeStr=boolean  SampleTime=1e-08
  Delay1 : Delay  DelayLength=double(1)  InitialCondition=0
  Multiport Switch : MultiPortSwitch  Inputs=6  DataPortForDefault=Additional data port  DiagnosticForDefault=None  SampleTime=1e-08  SaturateOnIntegerOverflow=off  InputSameDT=off
  WORDTOBOOL : Subsystem
  WORDTOBOOL_term{6..15} (10 alike) : Terminator
  ramwatcher : Subsystem
  valin : Outport  SampleTime=1e-08  InitialOutput=0
  wires:
  CLK/1 -> WORDTOBOOL/Trigger
  DATA/1 -> WORDTOBOOL/1(DATAIN)
  Constant3/1 -> Multiport Switch/8
  Multiport Switch/1 -> valin/1
  WORDTOBOOL/1(DATAOUT0) -> Multiport Switch/7
  WORDTOBOOL/2(DATAOUT1) -> Multiport Switch/6
  WORDTOBOOL/3(DATAOUT2) -> Multiport Switch/5
  WORDTOBOOL/4(DATAOUT3) -> Multiport Switch/4
  WORDTOBOOL/5(DATAOUT4) -> Multiport Switch/3
  WORDTOBOOL/6(DATAOUT5) -> Multiport Switch/2
  ramwatcher/1(SEL) -> Multiport Switch/1, Delay1/1
  WORDTOBOOL/7(DATAOUT6) -> WORDTOBOOL_term6/1
  WORDTOBOOL/8(DATAOUT7) -> WORDTOBOOL_term7/1
  WORDTOBOOL/9(DATAOUT8) -> WORDTOBOOL_term8/1
  WORDTOBOOL/10(DATAOUT9) -> WORDTOBOOL_term9/1
  WORDTOBOOL/11(DATAOUT10) -> WORDTOBOOL_term10/1
  WORDTOBOOL/12(DATAOUT11) -> WORDTOBOOL_term11/1
  WORDTOBOOL/13(DATAOUT12) -> WORDTOBOOL_term12/1
  WORDTOBOOL/14(DATAOUT13) -> WORDTOBOOL_term13/1
  WORDTOBOOL/15(DATAOUT14) -> WORDTOBOOL_term14/1
  WORDTOBOOL/16(DATAOUT15) -> WORDTOBOOL_term15/1
  Delay1/1 -> ramwatcher/1(In1)
  reset/1 -> ramwatcher/2(reset)
  SLOWCLCK/1 -> ramwatcher/Trigger

== system gm_UZ_EnDat/UZ_ENDAT/ageprovider/Detect Increase1 ==
  note: U(k)
  note: Edge
  U : Inport  OutDataTypeStr=boolean  SampleTime=1e-08
  FixPt Relational Operator : RelationalOperator  Operator=>  OutDataTypeStr=boolean  SampleTime=1e-08  InputSameDT=off
  rd_0 : Delay  DelayLength=double(1)  InitialCondition=0  SampleTime=1e-08
  t : hdlmdlgenlib/Buffer
  Y : Outport  SampleTime=1e-08
  wires:
  U/1 -> t/1, FixPt Relational Operator/1
  t/1 -> rd_0/1
  FixPt Relational Operator/1 -> Y/1
  rd_0/1 -> FixPt Relational Operator/2

== system gm_UZ_EnDat/UZ_ENDAT/ramselektor/Increment Stored Integer ==
  u : Inport  OutDataTypeStr=fixdt(0, 4, 0)
  FixPt Constant : Constant  OutDataTypeStr=fixdt(0, 4, 0)  SampleTime=-1
  FixPt Data Type Duplicate : DataTypeDuplicate  DisableCoverage=on  NumInputPorts=3
  FixPt Gateway In : DataTypeConversion  OutDataTypeStr=fixdt(0,4,0)
  FixPt Sum1 : Sum  OutDataTypeStr=fixdt(0, 4, 0)  AccumDataTypeStr=fixdt(0, 5, 0)
  sigspec : SignalSpecification  OutDataTypeStr=fixdt(0, 4, 0)  Dimensions=1
  y : Outport  InitialOutput=0
  wires:
  u/1 -> FixPt Sum1/1, FixPt Data Type Duplicate/2
  FixPt Constant/1 -> sigspec/1
  FixPt Gateway In/1 -> FixPt Sum1/2, FixPt Data Type Duplicate/3
  FixPt Sum1/1 -> FixPt Data Type Duplicate/1, y/1
  sigspec/1 -> FixPt Gateway In/1

== system gm_UZ_EnDat/UZ_ENDAT/signalquality/Detect Increase1 ==
  note: U(k)
  note: Edge
  U : Inport  OutDataTypeStr=boolean  SampleTime=1e-08
  FixPt Relational Operator : RelationalOperator  Operator=>  OutDataTypeStr=boolean  SampleTime=1e-08  InputSameDT=off
  rd_0 : Delay  DelayLength=double(1)  InitialCondition=0  SampleTime=1e-08
  t : hdlmdlgenlib/Buffer
  Y : Outport  SampleTime=1e-08
  wires:
  U/1 -> t/1, FixPt Relational Operator/1
  t/1 -> rd_0/1
  FixPt Relational Operator/1 -> Y/1
  rd_0/1 -> FixPt Relational Operator/2

== system gm_UZ_EnDat/UZ_ENDAT/timingprovider/CLKCNTER_POSCNTR ==
  CLK : Inport  OutDataTypeStr=boolean  PortDimensions=1  SampleTime=1e-08
  CLK2CNT : Inport  Port=2  OutDataTypeStr=boolean  PortDimensions=1  SampleTime=1e-08
  ResetCNT : Inport  Port=3  OutDataTypeStr=boolean  PortDimensions=1  SampleTime=1e-08
  Delay1 : Delay  DelayLength=double(1)  InitialCondition=0  SampleTime=1e-08
  Delay1_enbsw : Switch  Criteria=u2 ~= 0  Threshold=double(0)  OutDataTypeStr=uint32  SampleTime=1e-08  SaturateOnIntegerOverflow=off  InputSameDT=off
  Positional_Counter : Subsystem
  SetZero32modified : Subsystem
  SetZero32modified1 : Subsystem
  delayMatch : Delay  DelayLength=double(2)  InitialCondition=0  SampleTime=1e-08
  delayMatch1 : Delay  DelayLength=double(2)  InitialCondition=0  SampleTime=1e-08
  delayMatch2 : Delay  DelayLength=double(2)  InitialCondition=0  SampleTime=1e-08
  stateControl : Constant  OutDataTypeStr=boolean  SampleTime=1e-08
  CNT : Outport  SampleTime=1e-08
  wires:
  CLK/1 -> delayMatch/1
  CLK2CNT/1 -> delayMatch1/1
  stateControl/1 -> delayMatch2/1
  delayMatch2/1 -> Delay1_enbsw/2
  ResetCNT/1 -> SetZero32modified/2(setzero), SetZero32modified1/2(setzero)
  delayMatch/1 -> SetZero32modified/Trigger, SetZero32modified1/Trigger
  delayMatch1/1 -> Positional_Counter/Trigger
  SetZero32modified1/1(valueout) -> Positional_Counter/1(valueout)
  Positional_Counter/1(divider) -> SetZero32modified/1(valin)
  Delay1/1 -> Delay1_enbsw/3, SetZero32modified1/1(valin), CNT/1
  SetZero32modified/1(valueout) -> Delay1_enbsw/1
  Delay1_enbsw/1 -> Delay1/1

== system gm_UZ_EnDat/UZ_ENDAT/timingprovider/CLKCNTER_POSCNTR1 ==
  CLK : Inport  OutDataTypeStr=boolean  PortDimensions=1  SampleTime=1e-08
  CLK2CNT : Inport  Port=2  OutDataTypeStr=boolean  PortDimensions=1  SampleTime=1e-08
  ResetCNT : Inport  Port=3  OutDataTypeStr=boolean  PortDimensions=1  SampleTime=1e-08
  Delay1_enbsw : Switch  Criteria=u2 ~= 0  Threshold=double(0)  OutDataTypeStr=uint32  SampleTime=1e-08  SaturateOnIntegerOverflow=off  InputSameDT=off
  Positional_Counter : Subsystem
  SetZero32modified : Subsystem
  rd_0 : Delay  DelayLength=double(2)  InitialCondition=0  SampleTime=1e-08
  rd_1 : Delay  DelayLength=double(1)  InitialCondition=0  SampleTime=1e-08
  stateControl : Constant  OutDataTypeStr=boolean  SampleTime=1e-08
  CNT : Outport  SampleTime=1e-08
  wires:
  CLK/1 -> SetZero32modified/Trigger
  CLK2CNT/1 -> Positional_Counter/Trigger
  ResetCNT/1 -> SetZero32modified/2(setzero)
  stateControl/1 -> rd_0/1
  Positional_Counter/1(divider) -> SetZero32modified/1(valin)
  SetZero32modified/1(valueout) -> Delay1_enbsw/1
  rd_0/1 -> Delay1_enbsw/2
  Delay1_enbsw/1 -> rd_1/1
  rd_1/1 -> Delay1_enbsw/3, Positional_Counter/1(valueout), CNT/1

== system gm_UZ_EnDat/UZ_ENDAT/timingprovider/Compare To Constant ==
  u : Inport  OutDataTypeStr=uint32  SampleTime=1e-08
  Compare : RelationalOperator  Operator=>  OutDataTypeStr=boolean  SampleTime=1e-08
  Constant : Constant  Value=3  OutDataTypeStr=uint32  SampleTime=1e-08
  y : Outport  SampleTime=1e-08
  wires:
  u/1 -> Compare/1
  Compare/1 -> y/1
  Constant/1 -> Compare/2

== system gm_UZ_EnDat/UZ_ENDAT/timingprovider/Compare To Constant1 ==
  u : Inport  OutDataTypeStr=uint32  SampleTime=1e-08
  Compare : RelationalOperator  Operator===  OutDataTypeStr=boolean  SampleTime=1e-08
  Constant : Constant  Value=0  OutDataTypeStr=uint32  SampleTime=1e-08
  y : Outport  SampleTime=1e-08
  wires:
  u/1 -> Compare/1
  Compare/1 -> y/1
  Constant/1 -> Compare/2

== system gm_UZ_EnDat/UZ_ENDAT/timingprovider/Detect Increase1 ==
  note: U(k)
  note: Edge
  U : Inport  OutDataTypeStr=boolean  SampleTime=1e-08
  FixPt Relational Operator : RelationalOperator  Operator=>  OutDataTypeStr=boolean  SampleTime=1e-08  InputSameDT=off
  rd_0 : Delay  DelayLength=double(1)  InitialCondition=0  SampleTime=1e-08
  t : hdlmdlgenlib/Buffer
  Y : Outport  SampleTime=1e-08
  wires:
  U/1 -> t/1, FixPt Relational Operator/1
  t/1 -> rd_0/1
  FixPt Relational Operator/1 -> Y/1
  rd_0/1 -> FixPt Relational Operator/2

== system gm_UZ_EnDat/UZ_ENDAT/timingprovider/Subsystem2 ==
  elapsed : Inport  OutDataTypeStr=uint32  PortDimensions=1  SampleTime=1e-08
  clkcnt : Inport  Port=2  OutDataTypeStr=uint32  PortDimensions=1  SampleTime=1e-08
  Compare To Constant1 : Subsystem  mask(Compare To Constant){relop===, const=double(3), OutDataTypeStr=boolean, ZeroCross=on}
      mask prompts: relop "Simulink:masks:Operator_MP"; const "Simulink:masks:ConstantValue_MP"; OutDataTypeStr "Simulink:masks:OutputDataType_MP"; ZeroCross "Simulink:masks:EnableZerocrossingDetection_MP"
      mask help: Simulink:masks:CompareToConstant_MD
      mask init:
      | OutDataTypeStr = 'boolean';
      | ZeroCross = 'on';
      | blkName = 'UZ_EnDat/UZ_ENDAT/timingprovider/Subsystem2/Compare\nTo Constant1';
      | const = double(3);
      | const_str = '3';
      | const_val = double(3);
      | relop = '==';
      | setValue = 'boolean';
      | str = '== 3';
      mask TypeOptions relop: == | ~= | < | <= | >= | >
      mask TypeOptions OutDataTypeStr: Simulink:masks:uint8 | Simulink:masks:boolean
      mask Callback ZeroCross: sl('zeroCrossEnable', gcbh);
      mask Display: disp(str)
  Constant : Constant  Value=20  OutDataTypeStr=uint32  SampleTime=1e-08
  Delay1 : Delay  DelayLength=double(1)  InitialCondition=0  SampleTime=1e-08
  Delay1_enbsw : Switch  Criteria=u2 ~= 0  Threshold=double(0)  OutDataTypeStr=uint32  SampleTime=1e-08  SaturateOnIntegerOverflow=off  InputSameDT=off
  Detect Increase : Subsystem  mask(Detect Increase){vinit=double(0), InputProcessing=Elements as channels (sample based), OutDataTypeStr=boolean}
      mask prompts: vinit "Simulink:masks:InitialCondition_MP"; InputProcessing "Simulink:masks:InputProcessing_MP"; OutDataTypeStr "Simulink:masks:OutputDataType_MP"
      mask help: Simulink:masks:DetectIncrease_MD
      mask TypeOptions InputProcessing: Simulink:masks:ColumnsAsChannelsFrameBased | Simulink:masks:ElementsAsChannelsSampleBased
      mask TypeOptions OutDataTypeStr: Simulink:masks:uint8 | Simulink:masks:boolean
      mask Display: fprintf('U > U/z')
  HwModeRegister : Delay  DelayLength=double(1)  InitialCondition=0  SampleTime=1e-08
  HwModeRegister1 : Delay  DelayLength=double(1)  InitialCondition=0  SampleTime=1e-08
  PipelineRegister : Delay  DelayLength=double(1)  InitialCondition=0  SampleTime=1e-08
  Switch : Switch  Criteria=u2 > Threshold  Threshold=double(0)  OutDataTypeStr=uint32  SampleTime=1e-08  SaturateOnIntegerOverflow=off  InputSameDT=off
  delayMatch : Delay  DelayLength=double(2)  InitialCondition=0  SampleTime=1e-08
  nsproduct : Product  Inputs=**  OutDataTypeStr=fixdt(0, 64, 0)  SampleTime=1e-08
  nsproduct_out_dtc : DataTypeConversion  OutDataTypeStr=uint32  RndMeth=Simplest  SampleTime=1e-08
  stateControl : Constant  OutDataTypeStr=boolean  SampleTime=1e-08
  ns elapsed : Outport  SampleTime=1e-08
  wires:
  elapsed/1 -> Compare To Constant1/1(u)
  Compare To Constant1/1(y) -> Detect Increase/1(U)
  Constant/1 -> HwModeRegister/1
  nsproduct_out_dtc/1 -> ns elapsed/1
  PipelineRegister/1 -> nsproduct_out_dtc/1
  stateControl/1 -> delayMatch/1
  Switch/1 -> Delay1_enbsw/1, HwModeRegister1/1
  delayMatch/1 -> Delay1_enbsw/2
  clkcnt/1 -> Switch/1
  Detect Increase/1(Y) -> Switch/2
  Delay1/1 -> Delay1_enbsw/3, Switch/3
  Delay1_enbsw/1 -> Delay1/1
  nsproduct/1 -> PipelineRegister/1
  HwModeRegister/1 -> nsproduct/1
  HwModeRegister1/1 -> nsproduct/2

== system gm_UZ_EnDat/UZ_ENDAT/timingprovider/Subsystem3 ==
  elapsed : Inport  OutDataTypeStr=uint32  PortDimensions=1  SampleTime=1e-08
  clkcnt : Inport  Port=2  OutDataTypeStr=uint32  PortDimensions=1  SampleTime=1e-08
  Compare To Constant1 : Subsystem  mask(Compare To Constant){relop===, const=double(2), OutDataTypeStr=boolean, ZeroCross=on}
      mask prompts: relop "Simulink:masks:Operator_MP"; const "Simulink:masks:ConstantValue_MP"; OutDataTypeStr "Simulink:masks:OutputDataType_MP"; ZeroCross "Simulink:masks:EnableZerocrossingDetection_MP"
      mask help: Simulink:masks:CompareToConstant_MD
      mask init:
      | OutDataTypeStr = 'boolean';
      | ZeroCross = 'on';
      | blkName = 'UZ_EnDat/UZ_ENDAT/timingprovider/Subsystem3/Compare\nTo Constant1';
      | const = double(2);
      | const_str = '2';
      | const_val = double(2);
      | relop = '==';
      | setValue = 'boolean';
      | str = '== 2';
      mask TypeOptions relop: == | ~= | < | <= | >= | >
      mask TypeOptions OutDataTypeStr: Simulink:masks:uint8 | Simulink:masks:boolean
      mask Callback ZeroCross: sl('zeroCrossEnable', gcbh);
      mask Display: disp(str)
  Constant : Constant  Value=20  OutDataTypeStr=uint32  SampleTime=1e-08
  Delay1 : Delay  DelayLength=double(1)  InitialCondition=0  SampleTime=1e-08
  Delay1_enbsw : Switch  Criteria=u2 ~= 0  Threshold=double(0)  OutDataTypeStr=uint32  SampleTime=1e-08  SaturateOnIntegerOverflow=off  InputSameDT=off
  Detect Increase : Subsystem  mask(Detect Increase){vinit=double(0), InputProcessing=Elements as channels (sample based), OutDataTypeStr=boolean}
      mask prompts: vinit "Simulink:masks:InitialCondition_MP"; InputProcessing "Simulink:masks:InputProcessing_MP"; OutDataTypeStr "Simulink:masks:OutputDataType_MP"
      mask help: Simulink:masks:DetectIncrease_MD
      mask TypeOptions InputProcessing: Simulink:masks:ColumnsAsChannelsFrameBased | Simulink:masks:ElementsAsChannelsSampleBased
      mask TypeOptions OutDataTypeStr: Simulink:masks:uint8 | Simulink:masks:boolean
      mask Display: fprintf('U > U/z')
  HwModeRegister : Delay  DelayLength=double(1)  InitialCondition=0  SampleTime=1e-08
  HwModeRegister1 : Delay  DelayLength=double(1)  InitialCondition=0  SampleTime=1e-08
  PipelineRegister : Delay  DelayLength=double(1)  InitialCondition=0  SampleTime=1e-08
  Switch : Switch  Criteria=u2 > Threshold  Threshold=double(0)  OutDataTypeStr=uint32  SampleTime=1e-08  SaturateOnIntegerOverflow=off  InputSameDT=off
  delayMatch : Delay  DelayLength=double(2)  InitialCondition=0  SampleTime=1e-08
  nsproduct : Product  Inputs=**  OutDataTypeStr=fixdt(0, 64, 0)  SampleTime=1e-08
  nsproduct_out_dtc : DataTypeConversion  OutDataTypeStr=uint32  RndMeth=Simplest  SampleTime=1e-08
  stateControl : Constant  OutDataTypeStr=boolean  SampleTime=1e-08
  ns elapsed : Outport  SampleTime=1e-08
  wires:
  elapsed/1 -> Compare To Constant1/1(u)
  Compare To Constant1/1(y) -> Detect Increase/1(U)
  Constant/1 -> HwModeRegister/1
  nsproduct_out_dtc/1 -> ns elapsed/1
  PipelineRegister/1 -> nsproduct_out_dtc/1
  stateControl/1 -> delayMatch/1
  Switch/1 -> Delay1_enbsw/1, HwModeRegister1/1
  delayMatch/1 -> Delay1_enbsw/2
  clkcnt/1 -> Switch/1
  Detect Increase/1(Y) -> Switch/2
  Delay1/1 -> Delay1_enbsw/3, Switch/3
  Delay1_enbsw/1 -> Delay1/1
  nsproduct/1 -> PipelineRegister/1
  HwModeRegister/1 -> nsproduct/1
  HwModeRegister1/1 -> nsproduct/2

== system gm_UZ_EnDat/UZ_ENDAT/3timestorage/Triggered Subsystem/Counter Limited ==
  Force to be scalar : SignalSpecification  OutDataTypeStr=uint8  Dimensions=1
  Increment Real World : Subsystem  mask(Real World Value Increment){}
      mask help: Simulink:masks:RealWorldValueIncrement_MD
      mask Display: disp('V++')
  Output : Delay  DelayLength=double(1)  InitialCondition=0
  Wrap To Zero : Subsystem  mask(Wrap To Zero){Threshold=double(2)}
      mask prompts: Threshold "Simulink:masks:Threshold_MP"
      mask help: Simulink:masks:WrapToZero_MD
  sigspec : SignalSpecification  OutDataTypeStr=uint8  Dimensions=1
  y : Outport  InitialOutput=0
  wires:
  Output/1 -> y/1, Force to be scalar/1
  sigspec/1 -> Output/1
  Force to be scalar/1 -> Increment Real World/1(u)
  Increment Real World/1(y) -> Wrap To Zero/1(U)
  Wrap To Zero/1(Y) -> sigspec/1
